simulink model "Hbridge_PWM"  (R2020b)
settings: Solver=VariableStepAuto  StartTime=0.0  StopTime=0.02  RelTol=1e-3
libraries: powerlib x13, simulink x1
settings Model: Creator=Omar  LastModifiedBy=Omar
settings SolverCC: ZeroCrossAlgorithm=Adaptive
settings DataIOCC: ReturnWorkspaceOutputs=off
settings DebuggingCC: IgnoredZcDiagnostic=none

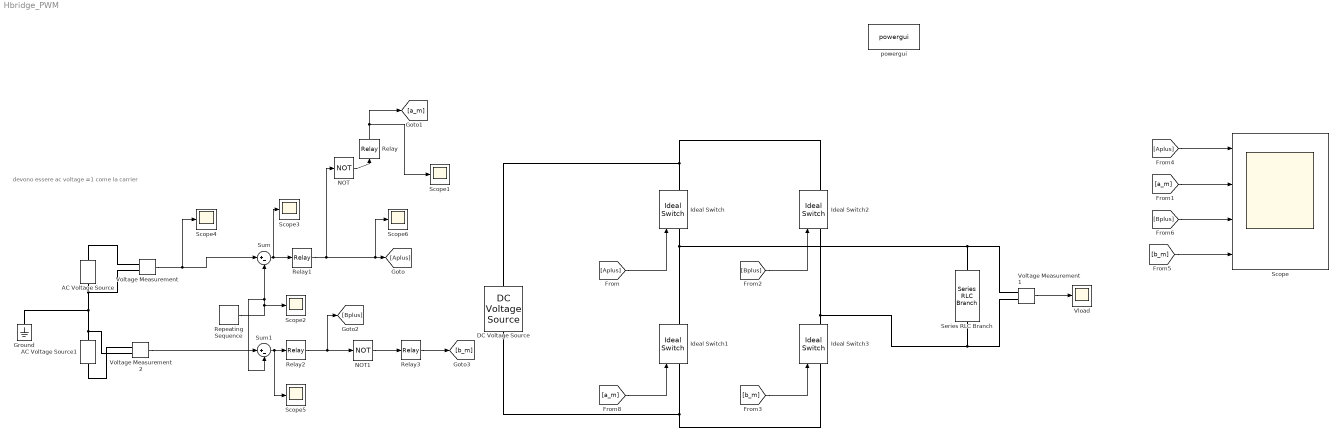
== system Hbridge_PWM ==
  note: devono essere ac voltage =1 come la carrier
  AC Voltage Source : powerlib/Electrical Sources/AC Voltage Source  Amplitude=1  Phase=0  Frequency=50  SampleTime=0  Measurements=None  BusType=swing  Pref=10e3  Qref=0  Qmin=-inf  Qmax=+inf
  AC Voltage Source1 : powerlib/Electrical Sources/AC Voltage Source  Amplitude=-1  Phase=0  Frequency=50  SampleTime=0  Measurements=None  BusType=swing  Pref=10e3  Qref=0  Qmin=-inf  Qmax=+inf
  DC Voltage Source : powerlib/Electrical Sources/DC Voltage Source  Amplitude=100  Measurements=None
  Ground : powerlib/Elements/Ground  LConnTagsString=a
  Ideal Switch{,1..3} (4 alike) : powerlib/Power Electronics/Ideal Switch  Ron=0.001  Lon=0  IC=0  Rs=1e5  Cs=inf  Measurements=on
  NOT : Logic  Operator=NOT  AllPortsSameDT=off  OutDataTypeStr=boolean
  NOT1 : Logic  Operator=NOT  IconShape=distinctive  AllPortsSameDT=off  OutDataTypeStr=boolean
  Relay{,1..3} (4 alike) : Relay
  Repeating Sequence : simulink/Sources/Repeating Sequence  rep_seq_t=[0 0.001/2 0.001]  rep_seq_y=[-1 1 -1]
  Scope : Scope  NumInputPorts=4
  Scope{1..6} (6 alike) : Scope
  Series RLC Branch : powerlib/Elements/Series RLC Branch  LConnTagsString=__new0  RConnTagsString=__new0  BranchType=R  Resistance=10  Inductance=10e-3  SetiL0=off  InitialCurrent=0  Capacitance=1e-6  Setx0=off  InitialVoltage=0  Measurements=None
  Sum : Sum  Inputs=|+-
  Sum1 : Sum  Inputs=|+-
  Vload : Scope
  Voltage Measurement : powerlib/Measurements/Voltage Measurement  PhasorSimulation=off  OutputType=Complex  PSBequivalent=0
  Voltage Measurement1 : powerlib/Measurements/Voltage Measurement  PhasorSimulation=off  OutputType=Complex  PSBequivalent=0
  Voltage Measurement2 : powerlib/Measurements/Voltage Measurement  PhasorSimulation=off  OutputType=Complex  PSBequivalent=0
  powergui : powerlib/powergui  Priority=1  SimulationMode=Discrete  SampleTime=1e-6  frequency=60  Iterations=50  frequencyindice=50  Pbase=100e6  ErrMax=1e-4  UnitsV=kV  UnitsW=MW  buscounter=0  FunctionMessages=off  echomessages=off  EnableUseOfTLC=off  CurrentSourceSwitches=off  DisableSnubberDevices=off  DisableRonSwitches=off  DisableVfSwitches=off  DisplayEquations=off  AutomaticDiscreteSolvers=off  SolverType=Tustin/Backward Euler (TBE)  Interpol=off  ExternalGateDelay=off  methode=off  Ts=100  x0status=blocks  SPID=on  SwTol=0  HookPort=off  NonlinearTolerance=1e-4  nMaxIteration=100  ContinueOnMaxIteration=off  RestoreLinks=warning  ResistiveCurrentMeasurement=off  Frange=[0:2:500]  Ylog=off  Xlog=on  ShowGrid=off  save=off  variable=ZData  structure=ScopeData2  ZoomFFT=off  StartTime=0  cycles=1  DisplayStyle=1  fundamental=50  FreqAxis=off  MaxFrequency=2500  frequencyindicesteady=1  RmsSteady=1  display=off
  wires:
  [Aplus] -> Ideal Switch/1
  [Bplus] -> Ideal Switch2/1
  [b_m] -> Scope/4
  Voltage Measurement1/1 -> Vload/1
  [a_m] -> Ideal Switch1/1
  [a_m] -> Scope/2
  [b_m] -> Ideal Switch3/1
  [Aplus] -> Scope/1
  [Bplus] -> Scope/3
  Voltage Measurement/1 -> Scope4/1, Sum/1
  Voltage Measurement2/1 -> Sum1/1
  Repeating Sequence/1 -> Sum1/2, Sum/2, Scope2/1
  NOT/1 -> Relay/1
  Sum/1 -> Scope3/1, Relay1/1
  Sum1/1 -> Scope5/1, Relay2/1
  Relay/1 -> Scope1/1, [a_m]
  Relay1/1 -> NOT/1, Scope6/1, [Aplus]
  Relay2/1 -> NOT1/1, [Bplus]
  NOT1/1 -> Relay3/1
  Relay3/1 -> [b_m]
  connections:
  Voltage Measurement1/LConn1 -- Ideal Switch/LConn1 -- Ideal Switch1/RConn1 -- Series RLC Branch/LConn1
  Ideal Switch2/RConn1 -- Ideal Switch/RConn1 -- DC Voltage Source/RConn1
  Ideal Switch1/LConn1 -- Ideal Switch3/LConn1 -- DC Voltage Source/LConn1
  Ideal Switch3/RConn1 -- Ideal Switch2/LConn1 -- Series RLC Branch/RConn1 -- Voltage Measurement1/LConn2
  AC Voltage Source1/LConn1 -- Voltage Measurement2/LConn2 -- Voltage Measurement/LConn2 -- AC Voltage Source/LConn1 -- Ground/LConn1
  AC Voltage Source/RConn1 -- Voltage Measurement/LConn1
  AC Voltage Source1/RConn1 -- Voltage Measurement2/LConn1
